simulink model "verify_PumpAdditionalIntegrationParallel_mdl_new"  (R2018b)
settings: Solver=ode45  StartTime=0.0  StopTime=400  MaxStep=5  RelTol=1e-3  EnableMultiTasking=on
undefined symbols (not defined in the file or in its folder): path_carnot
libraries: carnot x7, simulink x3
settings Model: Creator=drhf  LastModifiedBy=P41573
settings SolverCC: ZeroCrossAlgorithm=Adaptive
settings DataIOCC: SaveFormat=Array  SignalLoggingSaveFormat=ModelDataLogs
settings OptimizationCC: ExpressionDepthLimit=2147483647  LifeSpan=inf
settings DebuggingCC: UnderspecifiedInitializationDetection=Classic  MergeDetectMultiDrivingBlocksExec=none  SolverPrmCheckMsg=warning  StateNameClashWarn=warning  SFUnexpectedBacktrackingDiag=warning  SFNoUnconditionalDefaultTransitionDiag=warning  SFExecutionAtInitializationDiag=none
settings HardwareCC: ProdBitPerPointer=32  ProdBitPerSizeT=32  ProdBitPerPtrDiffT=32  ProdLargestAtomicFloat=None  ProdIntDivRoundTo=Undefined  ProdEndianess=Unspecified  ProdWordSize=32  ProdHWDeviceType=32-bit Generic
settings ModelReferenceCC: PropagateSignalLabelsOutOfModel=off
settings SFSimCC: SimUseLocalCustomCode=off
settings RTWCC: RTWUseLocalCustomCode=off
settings CodeAppCC: StateflowObjectComments=on
settings GRTTargetCC: TargetLangStandard=C89/C90 (ANSI)  GeneratePreprocessorConditionals=Disable all  CombineOutputUpdateFcns=off  GRTInterface=on
settings ConfigComp: CovMetricSettings=dw  CovHtmlReporting=on  CovSaveCumulativeToWorkspaceVar=on  CovSaveSingleToWorkspaceVar=on  CovExternalEMLEnable=off

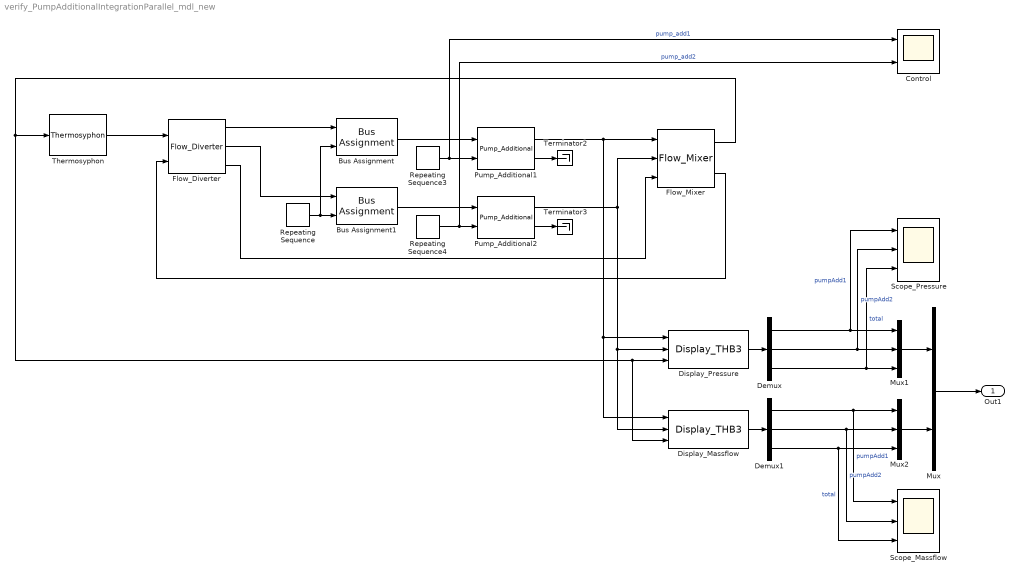
== system verify_PumpAdditionalIntegrationParallel_mdl_new ==
  Bus Assignment : BusAssignment  AssignedSignals=DPQuadratic
  Bus Assignment1 : BusAssignment  AssignedSignals=DPQuadratic
  Control : Scope  NumInputPorts=2
  Demux : Demux  Outputs=3
  Demux1 : Demux  Outputs=3
  Display_Massflow : carnot/Outputs/Display_THB3  t=off  m=on  p=off  id=off  mix=off  d=off
  Display_Pressure : carnot/Outputs/Display_THB3  t=off  m=off  p=on  id=off  mix=off  d=off
  Flow_Diverter : carnot/Hydraulics/Flow_Diverter
  Flow_Mixer : carnot/Hydraulics/Flow_Mixer
  Mux : Mux  Inputs=2
  Mux1 : Mux  Inputs=3
  Mux2 : Mux  Inputs=3
  Pump_Additional1 : carnot/Hydraulics/Pump_Additional  Tini=20  PathName=fullfile(path_carnot('libsl'), 'Hydraulics', 'Pump_Main', 'parameter_set')  FileName='Pump6m.mat'  userPath=off  userParam=off  a0=60000  a1=-43200  a2=0  dia=0.025  UA=1  mcp=4182  e0=50  e1=28.8  e2=-10.368
  Pump_Additional2 : carnot/Hydraulics/Pump_Additional  Tini=20  PathName=fullfile(path_carnot('libsl'), 'Hydraulics', 'Pump_Main', 'parameter_set')  FileName='Pump6m.mat'  userPath=off  userParam=off  a0=60000  a1=-43200  a2=0  dia=0.025  UA=1  mcp=4182  e0=50  e1=28.8  e2=-10.368
  Repeating Sequence : simulink/Sources/Repeating Sequence  rep_seq_t=[0 200 200.1 400]  rep_seq_y="[1e3 1e3 1e3 1e3]      % [0 0 1 1]*(6e4/0.01)^2"
  Repeating Sequence3 : simulink/Sources/Repeating Sequence  rep_seq_t=[0 40 40.1 50 60 200]  rep_seq_y=[1 1 0 0 1 1]
  Repeating Sequence4 : simulink/Sources/Repeating Sequence  rep_seq_t=[0 90 95 200]  rep_seq_y=[0 0 1 1]
  Scope_Massflow : Scope  NumInputPorts=3
  Scope_Pressure : Scope  NumInputPorts=3
  Terminator2 : Terminator
  Terminator3 : Terminator
  Thermosyphon : carnot/Hydraulics/Thermosyphon  p0=3e5  dia=0.025  fluid_id=Water  mix=0  mix2=0  mix3=0  t1=0.1
  Out1 : Outport  SampleTime=5
  wires:
  Pump_Additional1/2 -> Terminator2/1
  Bus Assignment/1 -> Pump_Additional1/1
  Display_Pressure/1 -> Demux/1
  Demux/1 -> Scope_Pressure/1, Mux1/1  "pumpAdd1"
  Demux/2 -> Scope_Pressure/2, Mux1/2  "pumpAdd2"
  Demux/3 -> Scope_Pressure/3, Mux1/3  "total"
  Repeating Sequence3/1 -> Control/1, Pump_Additional1/2  "pump_add1"
  Repeating Sequence/1 -> Bus Assignment/2, Bus Assignment1/2
  Pump_Additional2/2 -> Terminator3/1
  Bus Assignment1/1 -> Pump_Additional2/1
  Repeating Sequence4/1 -> Control/2, Pump_Additional2/2  "pump_add2"
  Pump_Additional2/1 -> Display_Massflow/2, Display_Pressure/2, Flow_Mixer/2
  Flow_Diverter/1 -> Bus Assignment/1
  Flow_Diverter/2 -> Bus Assignment1/1
  Flow_Diverter/3 -> Flow_Mixer/3
  Pump_Additional1/1 -> Display_Massflow/1, Display_Pressure/1, Flow_Mixer/1
  Flow_Mixer/2 -> Flow_Diverter/2
  Display_Massflow/1 -> Demux1/1
  Mux/1 -> Out1/1
  Demux1/1 -> Scope_Massflow/1, Mux2/1  "pumpAdd1"
  Demux1/2 -> Mux2/2, Scope_Massflow/2  "pumpAdd2"
  Demux1/3 -> Mux2/3, Scope_Massflow/3  "total"
  Mux1/1 -> Mux/1
  Mux2/1 -> Mux/2
  Flow_Mixer/1 -> Display_Massflow/3, Display_Pressure/3, Thermosyphon/1
  Thermosyphon/1 -> Flow_Diverter/1
